simulink model "cdg"  (Simulink 7.5)
settings: Solver=ode45  StartTime=0.0  StopTime=10.0  RelTol=1e-3
undefined symbols (not defined in the file or in its folder): magnitude, serial
libraries: dspxfrm3 x3, dspstat3 x2, instrumentlib x2, dspindex x2, dsparch4 x1, simulink_extras x1, commutil2 x1, dspswit3 x1, commseqgen2 x1, dspsigops x1
settings Model: Creator=sisa  LastModifiedBy=sisa  SimulationMode=external
settings OptimizationCC: OptimizeModelRefInitCode=on  LifeSpan=1
settings RTWCC: SystemTargetFile=ert.tlc  TemplateMakefile=ert_default_tmf  Description=Real-Time Workshop Embedded Coder  GenerateReport=on  ProcessScript=ert_make_rtw_hook  RTWUseSimCustomCode=on  IncludeHyperlinkInReport=on  LaunchReport=on  CheckMdlBeforeBuild=Warning
settings CodeAppCC: ForceParamTrailComments=on  IgnoreCustomStorageClasses=off
settings ERTTargetCC: MultiwordLength=2048  GenerateSampleERTMain=on  ERTCustomFileTemplate=example_file_process.tlc  ConvertIfToSwitch=off

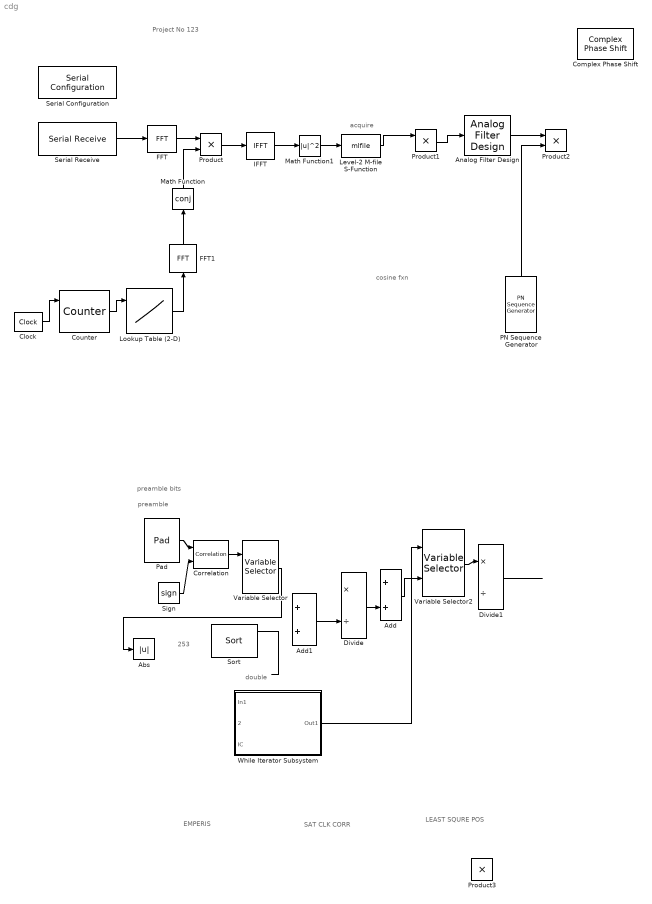
== system cdg ==
  note: Project No 123
  note: cosine fxn
  note: acquire
  note: 253
  note: double
  note: preamble
  note: preamble bits
  note: EMPERIS
  note: SAT CLK CORR
  note: LEAST SQURE POS
  Abs : Abs  OutDataType=fixdt(1, 16)  OutScaling=2^0
  Add : Sum  OutDataType=fixdt(1, 16)  OutScaling=2^-10
  Add1 : Sum  OutDataType=fixdt(1, 16)  OutScaling=2^-10
  Analog Filter Design : dsparch4/Analog Filter Design  method=Butterworth  filttype=Lowpass  N=8  Wlo=30  Whi=80  Rp=2  Rs=40
  Clock : simulink_extras/Flip Flops/Clock  SystemSampleTime=-1  MaskParam1=0.00000097752
  Complex Phase Shift : commutil2/Complex Phase Shift  SystemSampleTime=-1
  Correlation : dspstat3/Correlation  DialogController=dspDDGCreate  DialogControllerArgs=DataTag0  domain=Time  outputDataTypeStr=Inherit: Same as accumulator  outputLastDataTypeStr=Inherit: Same as accumulator  outputMin=[]  outputMax=[]  roundingMode=Floor  overflowMode=off
  Counter : dspswit3/Counter  Direction=Up  CountEvent=Either edge  CounterSize=User defined  MaxCount=1022  InitialCount=0  Output=Hit  HitValue=32  ResetInput=on  SamplesPerFrame=1  Ts=1  CntDtype=double  HitDtype=Logical
  Divide : Product  Inputs=*/  OutDataType=fixdt(1, 16)  OutScaling=2^-10
  Divide1 : Product  Inputs=*/  OutDataType=fixdt(1, 16)  OutScaling=2^-10
  FFT : dspxfrm3/FFT  DialogController=dspDDGCreate  DialogControllerArgs=DataTag1  CompMethod=Table lookup  TableOpt=NEW  TableOptActive=Speed  BitRevOrder=off  InheritFFTLength=on  FFTLength=64  SkipNorm=off  firstCoeffDataTypeStr=Inherit: Same word length as input  firstCoeffLastDataTypeStr=Inherit: Same word length as input  outputMin=[]  outputMax=[]  roundingMode=Floor  overflowMode=off
  FFT1 : dspxfrm3/FFT  DialogController=dspDDGCreate  DialogControllerArgs=DataTag2  CompMethod=Table lookup  TableOpt=NEW  TableOptActive=Speed  BitRevOrder=off  InheritFFTLength=on  FFTLength=64  SkipNorm=off  firstCoeffDataTypeStr=Inherit: Same word length as input  firstCoeffLastDataTypeStr=Inherit: Same word length as input  outputMin=[]  outputMax=[]  roundingMode=Floor  overflowMode=off
  IFFT : dspxfrm3/IFFT  DialogController=dspDDGCreate  DialogControllerArgs=DataTag3  CompMethod=Table lookup  TableOpt=NEW  TableOptActive=Speed  BitRevOrder=off  cs_in=off  SkipNorm=on  InheritFFTLength=on  FFTLength=64  mode=Complex  outSamplingMode=Sample based  firstCoeffDataTypeStr=Inherit: Same word length as input  firstCoeffLastDataTypeStr=Inherit: Same word length as input  outputMin=[]  outputMax=[]  roundingMode=Floor  overflowMode=off
  Level-2 M-file S-Function : M-S-Function
  Lookup Table (2-D) : Lookup2D  RowIndex=[1:3]  ColumnIndex=[1:3]  Table=[4 5 6;16 19 20;10 18 23]  OutDataType=fixdt(1, 16)  OutScaling=2^0
  Math Function : Math  Operator=conj  OutputSignalType=complex  OutDataType=fixdt(1, 16)  OutScaling=2^0  SaturateOnIntegerOverflow=on
  Math Function1 : Math  Operator=magnitude^2  OutputSignalType=real  OutDataType=fixdt(1, 16)  OutScaling=2^0  SaturateOnIntegerOverflow=on
  PN Sequence Generator : commseqgen2/PN Sequence Generator  poly=[1 0 0 0 0 1 1]  ini_sta=[0 0 0 0 0 1]  outBitMaskSource=Dialog parameter  shift=0  Ts=1  frameBased=off  sampPerFrame=1  reset=off  bitPackedOutputs=off  outDataType=double  numPackedBits=8  bitPackDataSigned=off  bitPackedOutDType=double
  Pad : dspsigops/Pad  padAlong=Columns  dimsToPad=1  valSrc=Specify via dialog  padVal=0  spec=Output size  padNumOutRowsSpecMethod=User-specified  numOutRows=1  padNumOutColsSpecMethod=User-specified  numOutCols=1  isVarDimsMode=off  padBeginning=0  padEnd=0  outSizeMode=User-specified  outSize=1  padSigAt=End  trunc_flag=None  roundingMode=Floor  overflowMode=off  truncOrWrapMode=Truncate  wrap_flag=None
  Product{,1..3} (4 alike) : Product  OutDataType=fixdt(1, 16)  OutScaling=2^0  RndMeth=Zero
  Serial Configuration : instrumentlib/Serial Configuration  Priority=-200000  DialogController=instrumentcreatedialog  DialogControllerArgs=DataTag4  ComPortMenu=COM1  ComPort=COM1  ObjConstructor=serial('COM1');  BaudRate=9600  DataBits=8  Parity=none  StopBits=1  FlowControl=none  Timeout=10  ByteOrder=LittleEndian
  Serial Receive : instrumentlib/Serial Receive  DialogController=instrumentcreatedialog  DialogControllerArgs=DataTag5  ComPortMenu=COM1  ComPort=COM1  ObjConstructor=serial('COM1');  Header=none  Terminator=<none>  DataSize="[1  1]"  DataType=uint8  EnableBlockingMode=on  ActionDataUnavailable=Output last received value  CustomValue=0  SampleTime=0.01
  Sign : Signum
  Sort : dspstat3/Sort  DialogController=dspDDGCreate  DialogControllerArgs=DataTag6  otype=Value and Index  dir=Ascending  sortAlg=Quick sort  accumDataTypeStr=Inherit: Same as product output  accumLastDataTypeStr=Inherit: Same as product output  roundingMode=Floor  overflowMode=off
  Variable Selector : dspindex/Variable Selector  NumInputs=1  rowsOrCols=Rows  IdxMode=Variable  Elements=[1 3]  ZerOneIdxMode=Zero-based  errmode=Clip and Warn  FillMode=on  FillValues=0
  Variable Selector2 : dspindex/Variable Selector  NumInputs=1  rowsOrCols=Rows  IdxMode=Variable  Elements=[1 3]  ZerOneIdxMode=One-based  errmode=Clip Index  FillMode=on  FillValues=0
  While Iterator Subsystem : Subsystem  TreatAsAtomicUnit=on
  wires:
  Serial Receive/1 -> FFT/1
  Product/1 -> IFFT/1
  FFT/1 -> Product/1
  Clock/1 -> Counter/1
  Counter/1 -> Lookup Table (2-D)/1
  Math Function/1 -> Product/2
  FFT1/1 -> Math Function/1
  Lookup Table (2-D)/1 -> FFT1/1
  IFFT/1 -> Math Function1/1
  ? -> Product1/2
  Analog Filter Design/1 -> Product2/1
  PN Sequence Generator/1 -> Product2/2
  Math Function1/1 -> Level-2 M-file S-Function/1
  Level-2 M-file S-Function/1 -> Product1/1
  Product1/1 -> Analog Filter Design/1
  ? -> Sign/1
  ? -> While Iterator Subsystem/2
  Pad/1 -> Correlation/1
  Sign/1 -> Correlation/2
  Correlation/1 -> Variable Selector/1
  Variable Selector/1 -> Abs/1
  ? -> Sort/1
  Sort/1 -> ?
  ? -> While Iterator Subsystem/1(In1)
  Add/1 -> Variable Selector2/2
  Add1/1 -> Divide/2
  Divide/1 -> Add/2
  Variable Selector2/1 -> Divide1/1
  Divide1/1 -> ?
  While Iterator Subsystem/1(Out1) -> Variable Selector2/1

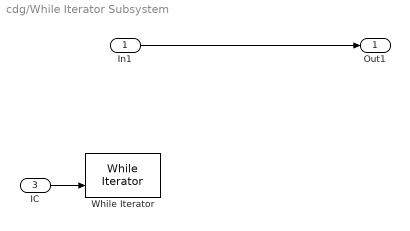
== system cdg/While Iterator Subsystem ==
  In1 : Inport  OutDataType=fixdt(1, 16)  OutScaling=2^0
  IC : Inport  Port=3  OutDataType=fixdt(1, 16)  OutScaling=2^0
  While Iterator : WhileIterator  ShowIterationPort=on
  Out1 : Outport  OutDataType=fixdt(1, 16)  OutScaling=2^0
  wires:
  IC/1 -> While Iterator/2
  In1/1 -> Out1/1
